simulink library "PDBHandler"  (R2016b)
settings: Solver=VariableStepAuto  StartTime=0.0  StopTime=10.0  RelTol=1e-3
settings Model: Creator=Nathan  LastModifiedBy=march

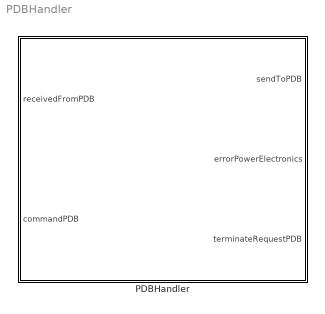
== system PDBHandler ==
  PDBHandler : Subsystem

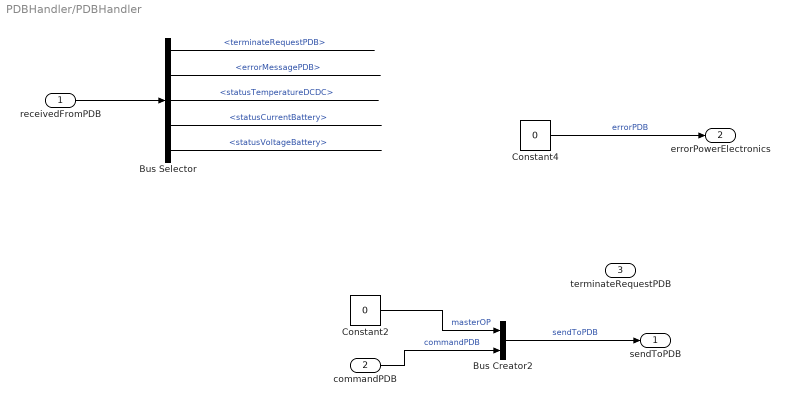
== system PDBHandler/PDBHandler ==
  receivedFromPDB : Inport  OutDataTypeStr=Bus: EtherCATReceivedFromPDB  BusOutputAsStruct=on
  commandPDB : Inport  Port=2
  Bus Creator2 : BusCreator  Inputs=2  OutDataTypeStr=Bus: EtherCATSendToPDB  NonVirtualBus=on
  Bus Selector : BusSelector  OutputSignals=terminateRequestPDB,errorMessagePDB,statusTemperatureDCDC,statusCurrentBattery,statusVoltageBattery
  Constant2 : Constant  Value=0
      settings: OpenFcn=|
      | b = get_param(gcb,'value');
      | if (strcmp(b,'1')),
      |   set_param (gcb,'value','0');
      | else
      |   set_param(gcb,'value','1');
      | end;
  Constant4 : Constant  Value=0
      settings: OpenFcn=|
      | b = get_param(gcb,'value');
      | if (strcmp(b,'72')),
      |   set_param (gcb,'value','0');
      | else
      |   set_param(gcb,'value','72');
      | end;
  sendToPDB : Outport  OutDataTypeStr=Bus: EtherCATSendToPDB
  errorPowerElectronics : Outport  Port=2
  terminateRequestPDB : Outport  Port=3
  wires:
  Bus Selector/5 -> ?  "<statusVoltageBattery>"
  Bus Selector/4 -> ?  "<statusCurrentBattery>"
  Bus Selector/3 -> ?  "<statusTemperatureDCDC>"
  Bus Selector/2 -> ?  "<errorMessagePDB>"
  Bus Selector/1 -> ?  "<terminateRequestPDB>"
  commandPDB/1 -> Bus Creator2/2  "commandPDB"
  receivedFromPDB/1 -> Bus Selector/1
  Bus Creator2/1 -> sendToPDB/1  "sendToPDB"
  Constant2/1 -> Bus Creator2/1  "masterOP"
  Constant4/1 -> errorPowerElectronics/1  "errorPDB"
